simulink library "ElectricalModelLib"  (R2019b)
settings: Solver=VariableStepAuto  StartTime=0.0  StopTime=10.0  RelTol=1e-3
libraries: $bdroot x2
settings Model: Creator=cleme  LastModifiedBy=cleme

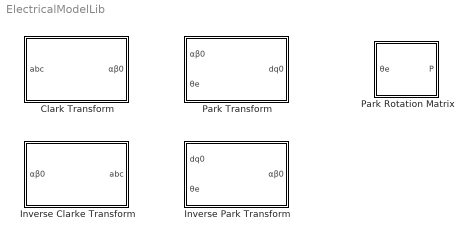
== system ElectricalModelLib ==
  Clark Transform : Subsystem  mask(ClarkTransform){}
      mask help:
      | Converts three-phases abc variables (separated by 120 electrical degrees) into two-phases αβ variables plus the zero component.
      |
      | For balanced three-phase variables, the zero component is equal to zero.
  Inverse Clarke Transform : Subsystem  mask(InverseClarkTransform){}
      mask help: Converts two-phases αβ0 variables into three-phases abc variables.
  Inverse Park Transform : Subsystem  mask(InverseParkTransform){}
      mask help:
      | Converts two-phases dq0  variables in the rotating frame into two-phases αβ0 variables in the stationnary frame.
      |
      | The α-axis and the q-axis are initially aligned.
  Park Rotation Matrix : Subsystem  mask(ParkRotationMatrix){}
      mask help:
      | Returns the rotation matrix to rotate a vector by θe from the stationnary αβ0 frame to the rotation dq0 frame.
      |
      | The q-axis is assumed to be aligned with the α when θe is zero.
  Park Transform : Subsystem  mask(ParkTransform){}
      mask help:
      | Converts two-phases αβ0 variables in the stationnary frame into two-phases dq0  variables in the rotating frame.
      |
      | The α-axis and the q-axis are initially aligned.

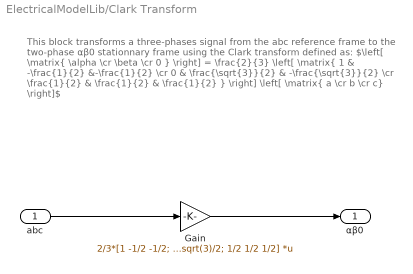
== system ElectricalModelLib/Clark Transform ==
  note: This block transforms a three-phases signal from the abc reference frame to the two-phase αβ0 stationnary frame using the Clark transform defined as:
      | $\left[ \matrix{ \alpha \cr \beta \cr 0 } \right] = \frac{2}{3} \left[ \matrix{ 1 & -\frac{1}{2} &-\frac{1}{2} \cr 0 & \frac{\sqrt{3}}{2} & -\frac{\sqrt{3}}{2} \cr \frac{1}{2} & \frac{1}{2} & \frac{1}{2} } \right] \left[ \matrix{ a \cr b \cr c} \right]$
  abc : Inport
  Gain : Gain  Gain=2/3*[1 -1/2 -1/2; 0 sqrt(3)/2 -sqrt(3)/2; 1/2 1/2 1/2]  Multiplication=Matrix(K*u)
  αβ0 : Outport
  wires:
  abc/1 -> Gain/1
  Gain/1 -> αβ0/1

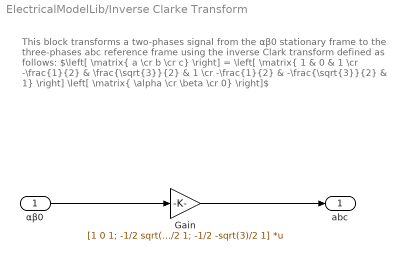
== system ElectricalModelLib/Inverse Clarke Transform ==
  note: This block transforms a two-phases signal from the αβ0 stationary frame to the three-phases abc reference frame using the inverse Clark transform defined as follows:
      | $\left[ \matrix{ a \cr b \cr c} \right] = \left[ \matrix{ 1 & 0 & 1 \cr -\frac{1}{2} & \frac{\sqrt{3}}{2} & 1 \cr -\frac{1}{2} & -\frac{\sqrt{3}}{2} & 1} \right] \left[ \matrix{ \alpha \cr \beta \cr 0} \right]$
  αβ0 : Inport
  Gain : Gain  Gain=[1 0 1; -1/2 sqrt(3)/2 1; -1/2 -sqrt(3)/2 1]  Multiplication=Matrix(K*u)
  abc : Outport
  wires:
  αβ0/1 -> Gain/1
  Gain/1 -> abc/1

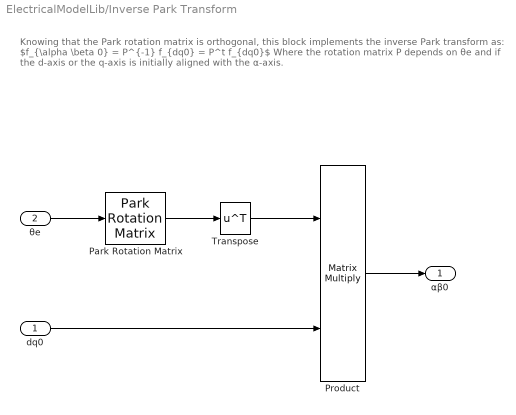
== system ElectricalModelLib/Inverse Park Transform ==
  note: Knowing that the Park rotation matrix is orthogonal, this block implements the inverse Park transform as:
      |
      | $f_{\alpha \beta 0} = P^{-1} f_{dq0} = P^t f_{dq0}$
      |
      | Where the rotation matrix P depends on θe and if the d-axis or the q-axis is initially aligned with the α-axis.
  dq0 : Inport
  θe : Inport  Port=2
  Park Rotation Matrix : $bdroot/Park Rotation Matrix
  Product : Product  Multiplication=Matrix(*)
  Transpose : Math  Operator=transpose  SaturateOnIntegerOverflow=on
  αβ0 : Outport
  wires:
  Transpose/1 -> Product/1
  dq0/1 -> Product/2
  Product/1 -> αβ0/1
  Park Rotation Matrix/1 -> Transpose/1
  θe/1 -> Park Rotation Matrix/1

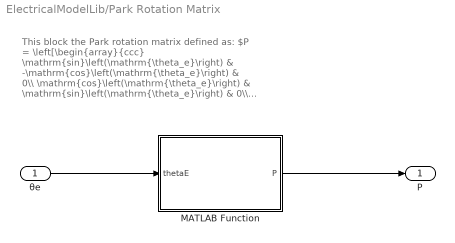
== system ElectricalModelLib/Park Rotation Matrix ==
  note: This block the Park rotation matrix defined as:
      | $P = \left[\begin{array}{ccc} \mathrm{sin}\left(\mathrm{\theta_e}\right) & -\mathrm{cos}\left(\mathrm{\theta_e}\right) & 0\\ \mathrm{cos}\left(\mathrm{\theta_e}\right) & \mathrm{sin}\left(\mathrm{\theta_e}\right) & 0\\ 0 & 0 & 1 \end{array}\right]$
  θe : Inport
  MATLAB Function : MATLAB Function  TreatAsAtomicUnit=on
  P : Outport
  wires:
  MATLAB Function/1(P) -> P/1
  θe/1 -> MATLAB Function/1(thetaE)

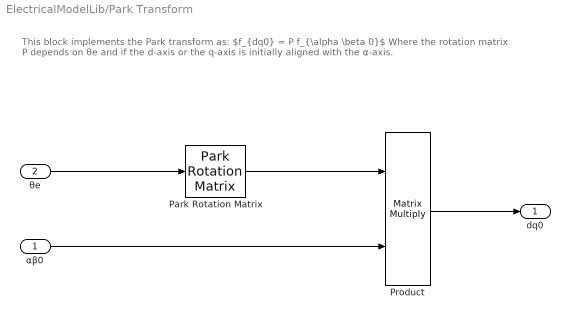
== system ElectricalModelLib/Park Transform ==
  note: This block implements the Park transform as:
      |
      | $f_{dq0} = P f_{\alpha \beta 0}$
      |
      | Where the rotation matrix P depends on θe and if the d-axis or the q-axis is initially aligned with the α-axis.
  αβ0 : Inport
  θe : Inport  Port=2
  Park Rotation Matrix : $bdroot/Park Rotation Matrix
  Product : Product  Multiplication=Matrix(*)
  dq0 : Outport
  wires:
  αβ0/1 -> Product/2
  Product/1 -> dq0/1
  θe/1 -> Park Rotation Matrix/1
  Park Rotation Matrix/1 -> Product/1

== matlab function ElectricalModelLib/Park Rotation Matrix/MATLAB Function ==
  data: thetaE input; P output
function P = getParkRotationMatrix(thetaE)

P = [sin(thetaE) -cos(thetaE) 0
    cos(thetaE) sin(thetaE) 0
    0 0 1];
